simulink model "GHV_open_VarialbeMass_trajectory_design_toolbox"  (R2023b)
settings: Solver=VariableStepAuto  StartTime=0.0  StopTime=10  FixedStep=0.0000001  MaxStep=0.001  RelTol=1e-3
InitFcn:
  | run('init.m')
undefined symbols (not defined in the file or in its folder): GHV_cfg
libraries: simulink_extras x3, aerolibtransform2 x3, aerolibasang x3, aerolibadyn x2, shared6dof x1, aerolibatmos2 x1
settings Model: SimulationMode=accelerator  Creator=Admin  LastModifiedBy=Admin
settings SolverCC: AllowMultiTaskInputOutput=on  ZeroCrossControl=EnableAll  ZeroCrossAlgorithm=Adaptive  AutoInsertRateTranBlk=on

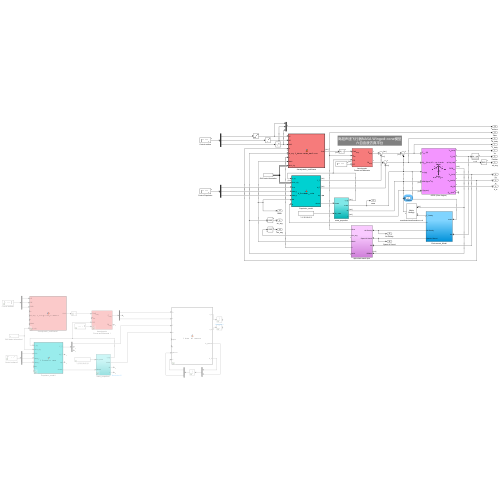
[thumbnail: Simulink's stored preview of the top-level diagram]
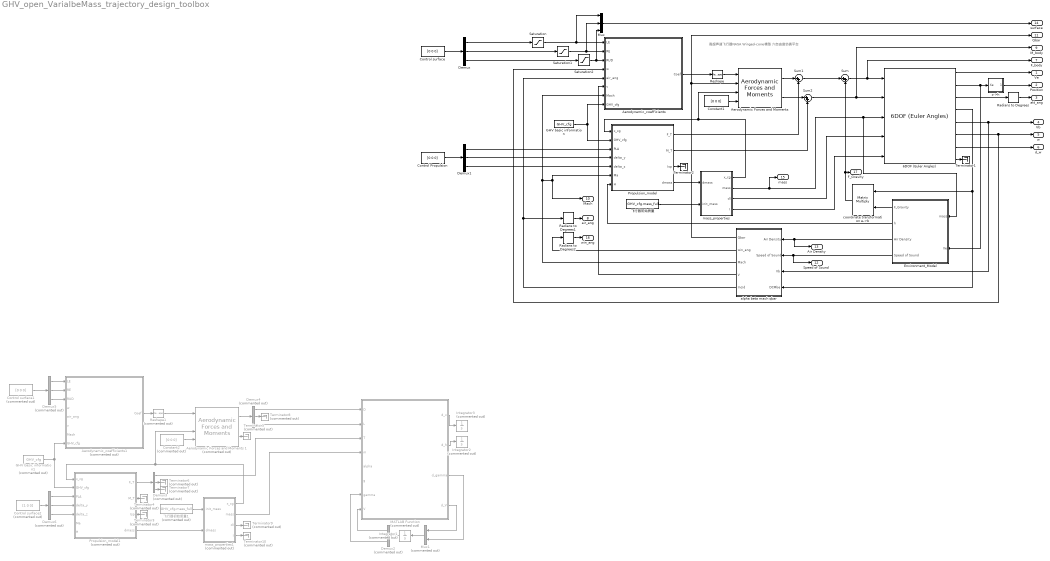
== system GHV_open_VarialbeMass_trajectory_design_toolbox ==
  note: 高超声速飞行器NASA Winged-cone模型
      | 六自由度仿真平台
  6DOF (Euler Angles) : shared6dof/6DOF (Euler Angles)  units=Metric (MKS)  mtype=Custom Variable  rep=Euler Angles  xme_0=Position_init  Vm_0=Speed_init  eul_0=Euler_init  pm_0=Omega_init  mass_0=GHV_cfg.mass_full  mass_e=0.5  mass_f=2.0  inertia=GHV_cfg.J  inertia_e=eye(3)  inertia_f=2*eye(3)  k_quat=1.0  vre_flag=off  abi_flag=off  aMode=0  xme_statename=''  Vm_statename=''  eul_statename=''  quat_statename=''  pm_statename=''  mass_statename=''
  "Aerodynamic Forces and Moments " : aerolibadyn/Aerodynamic Forces and Moments   inputAxes=Body  outputForceAxes=Body  outputMomentAxes=Body  S=GHV_cfg.s_ref  b=GHV_cfg.b_ref  cbar=GHV_cfg.c_ref
  Aerodynamic Forces and Moments 1 : aerolibadyn/Aerodynamic Forces and Moments   Commented=on  inputAxes=Body  outputForceAxes=Body  outputMomentAxes=Body  S=GHV_cfg.s_ref  b=GHV_cfg.b_ref  cbar=GHV_cfg.c_ref
  Aerodynamic_coefficients : MATLAB Function  TreatAsAtomicUnit=on
  Aerodynamic_coefficients1 : MATLAB Function  Commented=on  TreatAsAtomicUnit=on
  Constant1 : Constant  Value=[0 0 0]
  Constant2 : Constant  Commented=on  Value=[0 0 0]
  Control Propulsion : Constant  Value=[0 0 0]
  Control surface : Constant  Value=[0 0 0]
  Control surface1 : Constant  Commented=on  Value=[0 0 0]
  Control surface2 : Constant  Commented=on  Value=[1 0 0]
  Demux : Demux  Outputs=3
  Demux1 : Demux  Outputs=3
  Demux2 : Demux  Commented=on  Outputs=2
  Demux{3..6} (4 alike) : Demux  Commented=on  Outputs=3
  Environment_Model : Subsystem
  GHV basic information : Constant  Value=GHV_cfg  VectorParams1D=off  OutDataTypeStr=Bus: slBus1
  GHV basic information1 : Constant  Commented=on  Value=GHV_cfg  VectorParams1D=off  OutDataTypeStr=Bus: slBus1
  Integrator1 : Integrator  Commented=on
  Integrator2 : Integrator  Commented=on
  Integrator3 : Integrator  Commented=on
  MATLAB Function : MATLAB Function  Commented=on  TreatAsAtomicUnit=on
  Mux : Mux  Inputs=3
  Mux1 : Mux  Commented=on  Inputs=2
  Propulsion_model : MATLAB Function  TreatAsAtomicUnit=on
  Propulsion_model1 : MATLAB Function  Commented=on  TreatAsAtomicUnit=on
  Radians to Degrees : simulink_extras/Transformations/Radians to Degrees
  Radians to Degrees1 : simulink_extras/Transformations/Radians to Degrees
  Radians to Degrees2 : simulink_extras/Transformations/Radians to Degrees
  Reshape : Reshape
  Reshape1 : Reshape  Commented=on
  Saturation : Saturate  UpperLimit=30  LowerLimit=-30
  Saturation1 : Saturate  UpperLimit=30  LowerLimit=-30
  Saturation2 : Saturate  UpperLimit=30  LowerLimit=-30
  Sum : Sum  Inputs=|++
  Sum1 : Sum  Inputs=|++
  Sum2 : Sum  Inputs=|++
  Terminator1 : Terminator
  Terminator{3..10} (8 alike) : Terminator  Commented=on
  Terminator2 : Terminator
  alpha beta mach qbar : Subsystem
  coordinate transformation e->b : Product  Multiplication=Matrix(*)
  mass_properties : Subsystem
  mass_properties1 : Subsystem  Commented=on
  z->h : Subsystem
  飞行器初始质量 : Constant  Value=GHV_cfg.mass_full
  飞行器初始质量1 : Constant  Commented=on  Value=GHV_cfg.mass_full
  Ve : Outport
  Position : Outport  Port=2
  att_ang : Outport  Port=3
  Vb : Outport  Port=4
  w : Outport  Port=5
  d_w : Outport  Port=6
  F_body : Outport  Port=7
  air_ang : Outport  Port=8
  M_body : Outport  Port=9
  Mach : Outport  Port=10
  Qbar : Outport  Port=11
  Speed of Sound : Outport  Port=12
  Air Density : Outport  Port=13
  surface : Outport  Port=14
  mass : Outport  Port=15
  win_ang : Outport  Port=16
  F_Gravity : Outport  Port=17
  wires:
  "Aerodynamic Forces and Moments "/1 -> Sum1/1
  "Aerodynamic Forces and Moments "/2 -> Sum2/1
  Aerodynamic_coefficients/1(Coef) -> Reshape/1
  Environment_Model/1(F_Gravity) -> coordinate transformation e->b/2
  6DOF (Euler Angles)/4 -> alpha beta mach qbar/4(DCMbe), coordinate transformation e->b/1
  Sum/1 -> 6DOF (Euler Angles)/1, F_body/1
  coordinate transformation e->b/1 -> F_Gravity/1, Sum/2
  6DOF (Euler Angles)/2 -> Environment_Model/2(Xe), z->h/1(Xe)
  Environment_Model/4(Speed of Sound) -> alpha beta mach qbar/2(Speed of Sound), Speed of Sound/1
  Environment_Model/3(Air Density) -> alpha beta mach qbar/1(Air Density), Air Density/1
  6DOF (Euler Angles)/5 -> Vb/1, alpha beta mach qbar/3(Vb)
  alpha beta mach qbar/1(Qbar) -> "Aerodynamic Forces and Moments "/2, Qbar/1
  alpha beta mach qbar/5(Incid) -> Aerodynamic_coefficients/5(air_ang), Radians to Degrees1/1
  alpha beta mach qbar/4(V) -> Aerodynamic_coefficients/6(v)
  alpha beta mach qbar/3(Mach) -> Propulsion_model/6(Ma), Mach/1, Aerodynamic_coefficients/7(Mach)
  Constant1/1 -> "Aerodynamic Forces and Moments "/4
  6DOF (Euler Angles)/1 -> Ve/1
  6DOF (Euler Angles)/3 -> Radians to Degrees/1
  6DOF (Euler Angles)/7 -> d_w/1
  6DOF (Euler Angles)/8 -> Terminator1/1
  Control surface/1 -> Demux/1
  GHV basic information/1 -> Propulsion_model/2(GHV_cfg), Aerodynamic_coefficients/8(GHV_cfg)
  z->h/1(xyh) -> Position/1
  Radians to Degrees/1 -> att_ang/1
  Radians to Degrees1/1 -> air_ang/1
  Demux/1 -> Saturation/1
  Demux/2 -> Saturation1/1
  Demux/3 -> Saturation2/1
  6DOF (Euler Angles)/6 -> w/1, Aerodynamic_coefficients/4(w)
  Saturation/1 -> Mux/1, Aerodynamic_coefficients/1(LE)
  Saturation1/1 -> Mux/2, Aerodynamic_coefficients/2(RE)
  Saturation2/1 -> Mux/3, Aerodynamic_coefficients/3(RUD)
  Environment_Model/2(h) -> Propulsion_model/7(H)
  Control Propulsion/1 -> Demux1/1
  Demux1/1 -> Propulsion_model/3(PLA)
  Demux1/3 -> Propulsion_model/5(delta_z)
  Demux1/2 -> Propulsion_model/4(delta_y)
  飞行器初始质量/1 -> mass_properties/2(init_mass)
  Propulsion_model/4(dmass) -> mass_properties/1(dmass)
  mass_properties/2(mass) -> Environment_Model/1(mass), 6DOF (Euler Angles)/3, mass/1
  mass_properties/3(dI) -> 6DOF (Euler Angles)/4
  mass_properties/4(I) -> 6DOF (Euler Angles)/5
  mass_properties/1(x_cg) -> "Aerodynamic Forces and Moments "/3, Propulsion_model/1(x_cg)
  Sum1/1 -> Sum/1
  Sum2/1 -> 6DOF (Euler Angles)/2, M_body/1
  Propulsion_model/1(F_T) -> Sum1/2
  Propulsion_model/2(M_T) -> Sum2/2
  Propulsion_model/3(Isp) -> Terminator2/1
  Mux/1 -> surface/1
  alpha beta mach qbar/2(win_ang) -> Radians to Degrees2/1
  Reshape/1 -> "Aerodynamic Forces and Moments "/1
  Radians to Degrees2/1 -> win_ang/1
  Mux1/1 -> Integrator1/1
  Integrator1/1 -> Demux2/1
  MATLAB Function/4(d_V) -> Mux1/1
  Demux2/1 -> MATLAB Function/8(V)
  MATLAB Function/3(d_gamma) -> Mux1/2
  Demux2/2 -> MATLAB Function/7(gamma)
  MATLAB Function/2(d_h) -> Integrator2/1
  MATLAB Function/1(d_x) -> Integrator3/1
  Aerodynamic_coefficients1/1(Coef) -> Reshape1/1
  Propulsion_model1/4(dmass) -> mass_properties1/2(dmass)
  Reshape1/1 -> Aerodynamic Forces and Moments 1/1
  mass_properties1/1(x_cg) -> Propulsion_model1/1(x_cg), Aerodynamic Forces and Moments 1/3
  Constant2/1 -> Aerodynamic Forces and Moments 1/4
  Propulsion_model1/3(Isp) -> Terminator3/1
  Propulsion_model1/2(M_T) -> Terminator4/1
  Aerodynamic Forces and Moments 1/2 -> Terminator5/1
  Propulsion_model1/1(F_T) -> Demux3/1
  Demux3/2 -> Terminator6/1
  Demux3/3 -> Terminator7/1
  Demux3/1 -> MATLAB Function/3(T)
  Aerodynamic Forces and Moments 1/1 -> Demux4/1
  Demux4/2 -> Terminator8/1
  Demux4/1 -> MATLAB Function/1(D)
  Demux4/3 -> MATLAB Function/2(L)
  mass_properties1/2(mass) -> MATLAB Function/4(m)
  mass_properties1/3(dI) -> Terminator9/1
  mass_properties1/4(I) -> Terminator10/1
  飞行器初始质量1/1 -> mass_properties1/1(init_mass)
  GHV basic information1/1 -> Aerodynamic_coefficients1/8(GHV_cfg), Propulsion_model1/2(GHV_cfg)
  Demux5/3 -> Aerodynamic_coefficients1/3(RUD)
  Demux5/1 -> Aerodynamic_coefficients1/1(LE)
  Demux5/2 -> Aerodynamic_coefficients1/2(RE)
  Control surface1/1 -> Demux5/1
  Control surface2/1 -> Demux6/1
  Demux6/1 -> Propulsion_model1/3(PLA)
  Demux6/2 -> Propulsion_model1/4(delta_y)
  Demux6/3 -> Propulsion_model1/5(delta_z)

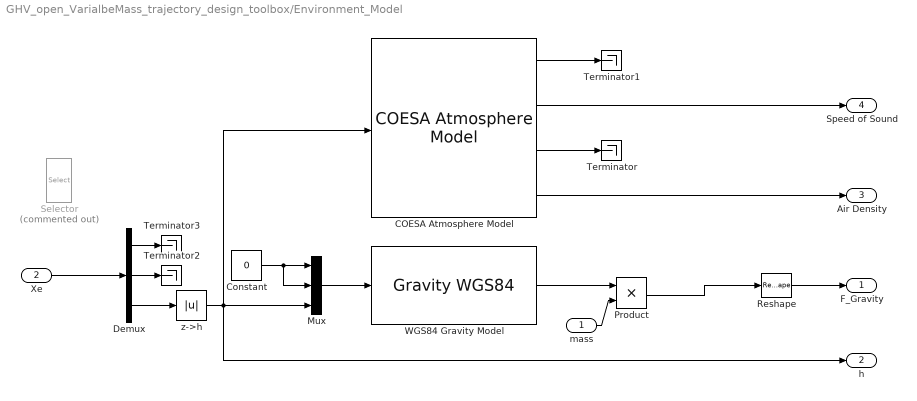
== system GHV_open_VarialbeMass_trajectory_design_toolbox/Environment_Model ==
  mass : Inport
  Xe : Inport  Port=2
  COESA Atmosphere Model : aerolibatmos2/COESA Atmosphere Model  units=Metric (MKS)  spec=1976 COESA-extended U.S. Standard Atmosphere  model=Profile  profile_var=High temperature  profile_percent=1%  profile_alt=5 km (16404 ft)  envelope_var=High temperature  envelope_percent=1%  action=Warning
  Constant : Constant  Value=0
  Demux : Demux  Outputs=3
  Mux : Mux  Inputs=3
  Product : Product
  Reshape : Reshape
  Selector : Selector  Commented=on  InputPortWidth=3  IndexOptions=Index vector (dialog)  Indices=[3]  OutputSizes=1
  Terminator{,1..3} (4 alike) : Terminator
  "WGS84 Gravity Model  " : GravityWGS84  action=None
  z->h : Abs  SaturateOnIntegerOverflow=off
  F_Gravity : Outport
  h : Outport  Port=2
  Air Density : Outport  Port=3
  Speed of Sound : Outport  Port=4
  wires:
  Product/1 -> Reshape/1
  Constant/1 -> Mux/2, Mux/1
  z->h/1 -> h/1, COESA Atmosphere Model/1, Mux/3
  Mux/1 -> "WGS84 Gravity Model  "/1
  COESA Atmosphere Model/1 -> Terminator1/1
  COESA Atmosphere Model/2 -> Speed of Sound/1
  COESA Atmosphere Model/3 -> Terminator/1
  "WGS84 Gravity Model  "/1 -> Product/1
  COESA Atmosphere Model/4 -> Air Density/1
  Reshape/1 -> F_Gravity/1
  Xe/1 -> Demux/1
  Demux/3 -> z->h/1
  Demux/2 -> Terminator2/1
  Demux/1 -> Terminator3/1
  mass/1 -> Product/2

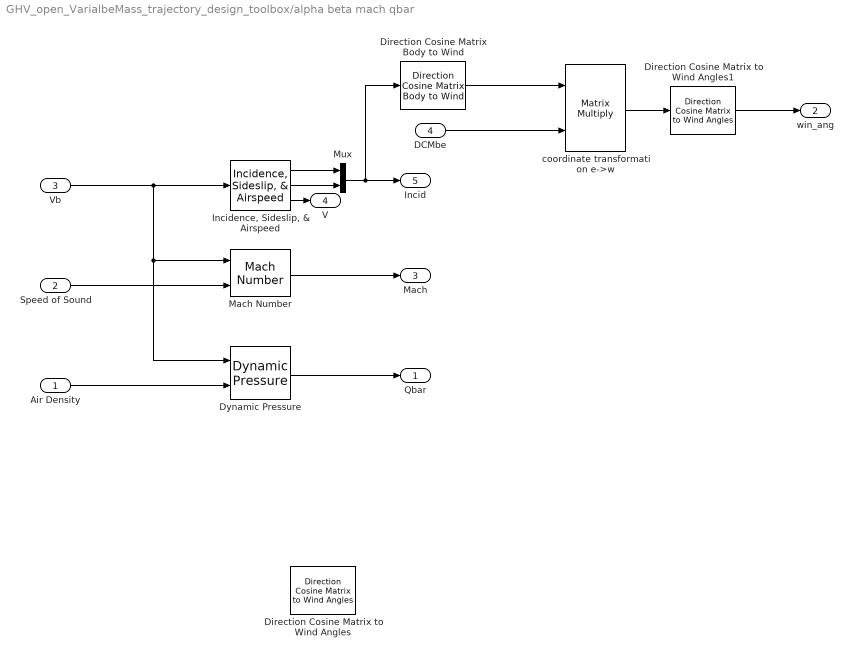
== system GHV_open_VarialbeMass_trajectory_design_toolbox/alpha beta mach qbar ==
  Air Density : Inport
  Speed of Sound : Inport  Port=2
  Vb : Inport  Port=3
  DCMbe : Inport  Port=4
  Direction Cosine Matrix Body to Wind : aerolibtransform2/Direction Cosine Matrix Body to Wind
  Direction Cosine Matrix to Wind Angles : aerolibtransform2/Direction Cosine Matrix to Wind Angles  action=None  tolerance=eps(2)
  Direction Cosine Matrix to Wind Angles1 : aerolibtransform2/Direction Cosine Matrix to Wind Angles  action=None  tolerance=eps(2)
  Dynamic Pressure : aerolibasang/Dynamic Pressure
  "Incidence, Sideslip, & Airspeed" : aerolibasang/Incidence, Sideslip, & Airspeed
  Mach Number : aerolibasang/Mach Number
  Mux : Mux  Inputs=2
  coordinate transformation e->w : Product  Multiplication=Matrix(*)
  Qbar : Outport
  win_ang : Outport  Port=2
  Mach : Outport  Port=3
  V : Outport  Port=4
  Incid : Outport  Port=5
  wires:
  Speed of Sound/1 -> Mach Number/2
  Mach Number/1 -> Mach/1
  "Incidence, Sideslip, & Airspeed"/2 -> Mux/2
  Vb/1 -> Dynamic Pressure/1, Mach Number/1, "Incidence, Sideslip, & Airspeed"/1
  Dynamic Pressure/1 -> Qbar/1
  Mux/1 -> Direction Cosine Matrix Body to Wind/1, Incid/1
  "Incidence, Sideslip, & Airspeed"/1 -> Mux/1
  Air Density/1 -> Dynamic Pressure/2
  "Incidence, Sideslip, & Airspeed"/3 -> V/1
  DCMbe/1 -> coordinate transformation e->w/2
  Direction Cosine Matrix Body to Wind/1 -> coordinate transformation e->w/1
  coordinate transformation e->w/1 -> Direction Cosine Matrix to Wind Angles1/1
  Direction Cosine Matrix to Wind Angles1/1 -> win_ang/1

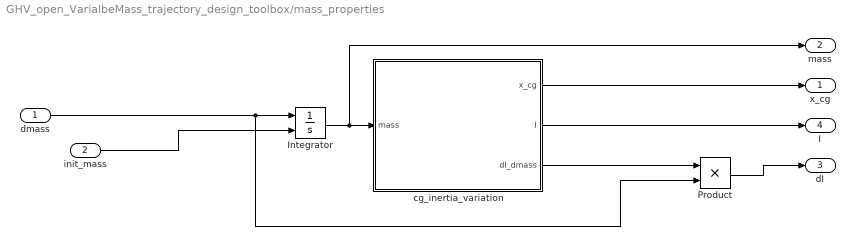
== system GHV_open_VarialbeMass_trajectory_design_toolbox/mass_properties ==
  dmass : Inport
  init_mass : Inport  Port=2
  Integrator : Integrator  InitialConditionSource=external
  Product : Product
  cg_inertia_variation : MATLAB Function  TreatAsAtomicUnit=on
  x_cg : Outport
  mass : Outport  Port=2
  dI : Outport  Port=3
  I : Outport  Port=4
  wires:
  Integrator/1 -> mass/1, cg_inertia_variation/1(mass)
  init_mass/1 -> Integrator/2
  cg_inertia_variation/3(dI_dmass) -> Product/1
  dmass/1 -> Product/2, Integrator/1
  cg_inertia_variation/2(I) -> I/1
  cg_inertia_variation/1(x_cg) -> x_cg/1
  Product/1 -> dI/1

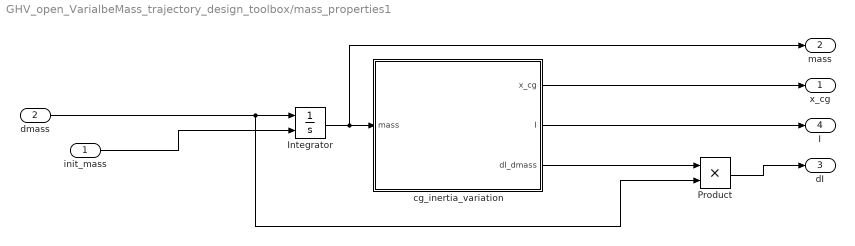
== system GHV_open_VarialbeMass_trajectory_design_toolbox/mass_properties1 ==
  init_mass : Inport
  dmass : Inport  Port=2
  Integrator : Integrator  InitialConditionSource=external
  Product : Product
  cg_inertia_variation : MATLAB Function  TreatAsAtomicUnit=on
  x_cg : Outport
  mass : Outport  Port=2
  dI : Outport  Port=3
  I : Outport  Port=4
  wires:
  Integrator/1 -> mass/1, cg_inertia_variation/1(mass)
  init_mass/1 -> Integrator/2
  cg_inertia_variation/3(dI_dmass) -> Product/1
  dmass/1 -> Product/2, Integrator/1
  cg_inertia_variation/2(I) -> I/1
  cg_inertia_variation/1(x_cg) -> x_cg/1
  Product/1 -> dI/1

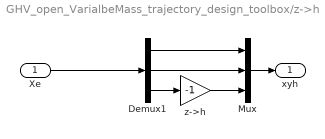
== system GHV_open_VarialbeMass_trajectory_design_toolbox/z->h ==
  Xe : Inport
  Demux1 : Demux  Outputs=3
  Mux : Mux  Inputs=3
  z->h : Gain  Gain=-1
  xyh : Outport
  wires:
  z->h/1 -> Mux/3
  Demux1/2 -> Mux/2
  Demux1/3 -> z->h/1
  Demux1/1 -> Mux/1
  Xe/1 -> Demux1/1
  Mux/1 -> xyh/1

== matlab function GHV_open_VarialbeMass_trajectory_design_toolbox/mass_properties1/cg_inertia_variation ==
  data: mass input; x_cg output; I output; dI_dmass output
function [x_cg, I, dI_dmass] = S_cg_inertia_variation(mass)

     [x_cg, I, dI_dmass] = cg_inertia_variation(mass);
     
end

== matlab function GHV_open_VarialbeMass_trajectory_design_toolbox/Propulsion_model ==
  data: x_cg input; GHV_cfg input; PLA input; delta_y input; delta_z input; Ma input; H input; F_T output; M_T output; Isp output; dmass output
function  [F_T, M_T, Isp, dmass] = S_Propulsion_model(x_cg, GHV_cfg, PLA, delta_y, delta_z, Ma, H)
    F_T = zeros(3, 1); %#ok<PREALL>
    M_T = zeros(3, 1); %#ok<PREALL>
   [F_T, M_T, Isp, dmass] = Propulsion_model(PLA, H, Ma, delta_y, delta_z, GHV_cfg, x_cg);

end

== matlab function GHV_open_VarialbeMass_trajectory_design_toolbox/Aerodynamic_coefficients ==
  data: LE input; Coef output; RE input; RUD input; w input; air_ang input; v input; Mach input; GHV_cfg input
function Coef = S_Aerodynamic_coefficients(LE, RE, RUD, w, air_ang,v, Mach, GHV_cfg)
    Coef = zeros(6, 1);
    Coef = Aerodynamic_coefficients(LE, RE, RUD, air_ang, v, w, Mach, GHV_cfg);

end

== matlab function GHV_open_VarialbeMass_trajectory_design_toolbox/mass_properties/cg_inertia_variation ==
  data: mass input; x_cg output; I output; dI_dmass output
function [x_cg, I, dI_dmass] = S_cg_inertia_variation(mass)

     [x_cg, I, dI_dmass] = cg_inertia_variation(mass);
     
end

== matlab function GHV_open_VarialbeMass_trajectory_design_toolbox/MATLAB Function ==
  data: D input; L input; d_x output; d_h output; d_gamma output; T input; m input; d_V output; alpha input; g input; gamma input; V input
function [d_x, d_h, d_gamma, d_V] = S_three_dof_trajectory(D, L, T, m, alpha, g, gamma, V)

    [d_V, d_gamma, d_x, d_h] = three_dof_trajectory(T, D, L, alpha, m, g, V, gamma);


end

== matlab function GHV_open_VarialbeMass_trajectory_design_toolbox/Aerodynamic_coefficients1 ==
  data: LE input; Coef output; RE input; RUD input; w input; air_ang input; v input; Mach input; GHV_cfg input
function Coef = S_Aerodynamic_coefficients(LE, RE, RUD, w, air_ang,v, Mach, GHV_cfg)
    Coef = zeros(6, 1);
    Coef = Aerodynamic_coefficients(LE, RE, RUD, air_ang, v, w, Mach, GHV_cfg);

end

== matlab function GHV_open_VarialbeMass_trajectory_design_toolbox/Propulsion_model1 ==
  data: x_cg input; GHV_cfg input; PLA input; delta_y input; delta_z input; Ma input; H input; F_T output; M_T output; Isp output; dmass output
function  [F_T, M_T, Isp, dmass] = S_Propulsion_model(x_cg, GHV_cfg, PLA, delta_y, delta_z, Ma, H)
    F_T = zeros(3, 1); %#ok<PREALL>
    M_T = zeros(3, 1); %#ok<PREALL>
   [F_T, M_T, Isp, dmass] = Propulsion_model(PLA, H, Ma, delta_y, delta_z, GHV_cfg, x_cg);

end
